simulink model "Rigid_Body_control"  (R2016a)
settings: Solver=VariableStepAuto  StartTime=0.0  StopTime=100  RelTol=1e-3
values from neighbouring files (symbols this model uses):
  kd = 2*z*wn    (= 0.068)    [Dynamic_Dependant_control.m]
  kp = wn.^2    [Dynamic_Dependant_control.m]
libraries: lib_exmp x1
settings Model: Creator=devantormey  LastModifiedBy=devantormey

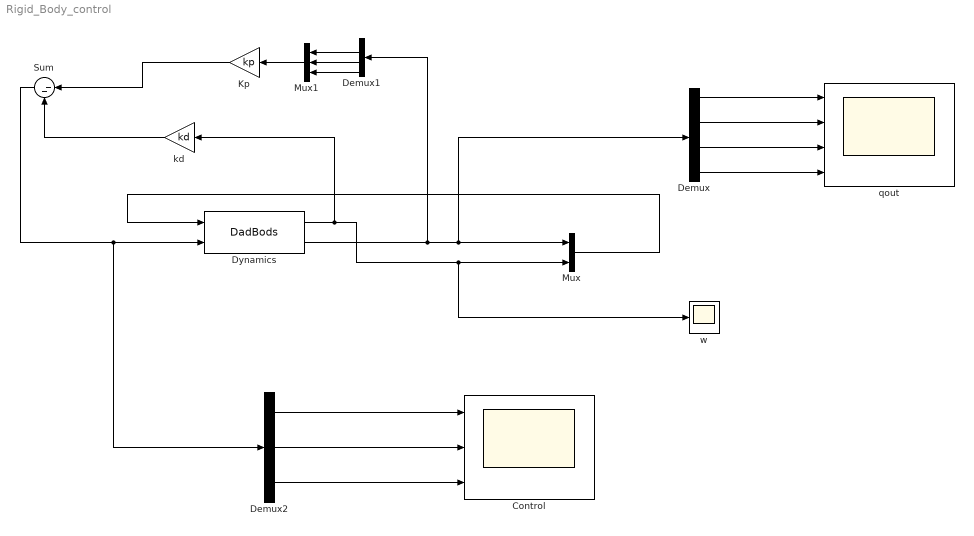
== system Rigid_Body_control ==
  Control : Scope  NumInputPorts=3
  Demux : Demux
  Demux1 : Demux
  Demux2 : Demux  Outputs=3
  "Dynamics " : lib_exmp/DadBods 
  Kp : Gain  Gain=kp
  Mux : Mux  Inputs=2
  Mux1 : Mux  Inputs=3
  Sum : Sum  Inputs=|--
  kd : Gain  Gain=kd
  qout : Scope  NumInputPorts=4
  w : Scope
  wires:
  "Dynamics "/2 -> Demux1/1, Demux/1, Mux/1
  Mux/1 -> "Dynamics "/1
  Demux/1 -> qout/1
  Demux/2 -> qout/2
  Demux/3 -> qout/3
  Demux/4 -> qout/4
  "Dynamics "/1 -> kd/1, w/1, Mux/2
  kd/1 -> Sum/2
  Sum/1 -> Demux2/1, "Dynamics "/2
  Mux1/1 -> Kp/1
  Demux1/2 -> Mux1/1
  Demux1/3 -> Mux1/2
  Demux1/4 -> Mux1/3
  Demux2/2 -> Control/2
  Demux2/1 -> Control/1
  Demux2/3 -> Control/3
  Kp/1 -> Sum/1
